simulink model "TCP_Test"  (R2024a)
settings: Solver=FixedStepAuto  StartTime=0.0  StopTime=10.0  RelTol=1e-3  EnableMultiTasking=on
libraries: px4Sensorslib x1, px4Utilslib x1
settings Model: ExtModeTrigDuration=10  Creator=root  LastModifiedBy=root
settings SolverCC: PositivePriorityOrder=on
settings OptimizationCC: OptimizeBlockIOStorage=off  BufferReuse=off  ReuseModelBlockBuffer=off  GlobalBufferReuse=off  ExpressionFolding=off  EnableMemcpy=off  PassReuseOutputArgsAs=Individual arguments  LocalBlockOutputs=off  ZeroExternalMemoryAtStartup=off  ZeroInternalMemoryAtStartup=off  MaxStackSize=64  OptimizeDataStoreBuffers=off  BusAssignmentInplaceUpdate=off  OptimizationLevel=level0  OptimizationCustomize=off  EfficientTunableParamExpr=on
settings DebuggingCC: ParameterTunabilityLossMsg=error
settings HardwareCC: ProdBitPerPointer=32  ProdBitPerSizeT=32  ProdBitPerPtrDiffT=32  ProdLargestAtomicInteger=Long  ProdLargestAtomicFloat=Double  ProdWordSize=32  ProdLongLongMode=on  ProdHWDeviceType=ARM Compatible->ARM Cortex
settings SFSimCC: SimUserSources=tcp_send.c  SimUserIncludeDirs=/home/judson/Desktop/Pixhawk/MATLAB/TCP_Test  MATLABDynamicMemAlloc=off  SimTargetLang=C++
settings SFSimCC: SimCustomHeaderCode=|
  | #include "tcp_send.h"
  | #include <netinet/in.h>
  | #include <sys/types.h>
  | #include <sys/socket.h>
  | #include <arpa/inet.h>
  | #include <errno.h>
  | #include <stdio.h>
  | #include <string.h>
  | #include <unistd.h>
settings RTWCC: Description=Embedded Coder  SystemTargetFile=ert.tlc  HardwareBoard=PX4 Pixhawk 6x  TLCOptions="-aInlineSetEventsForThisBaseRateFcn=TLC_FALSE -aSuppressMultiTaskScheduler=TLC_FALSE  -aRateBasedStepFcn=0"  TemplateMakefile=ert_default_tmf  RTWUseSimCustomCode=on  CustomInclude=/home/judson/Desktop/Pixhawk/MATLAB/TCP_Test  CustomSource=tcp_send.c  Toolchain=GNU Tools for PX4 Autopilots  BuildConfiguration=Debug  TargetLang=C++
settings RTWCC: CustomHeaderCode=|
  | #include "tcp_send.h"
  | #include <netinet/in.h>
  | #include <sys/types.h>
  | #include <sys/socket.h>
  | #include <arpa/inet.h>
  | #include <errno.h>
  | #include <stdio.h>
  | #include <string.h>
  | #include <unistd.h>
settings CodeAppCC: ForceParamTrailComments=on  IgnoreCustomStorageClasses=off  OperatorAnnotations=on  SimulinkDataObjDesc=on  SFDataObjDesc=on  MATLABFcnDesc=on  InsertBlockDesc=on  MATLABSourceComments=on  EnableCustomComments=on  ReqsInCode=on
settings ERTTargetCC: TargetLangStandard=C++11 (ISO)  SupportNonFinite=off  ExtModeTransport=3  ExtModeStaticAlloc=on  ExtModeStaticAllocSize=1024  ExtModeMexFile=ext_xcp  ExtModeIntrfLevel=Level2 - Open  PreserveIfCondition=on

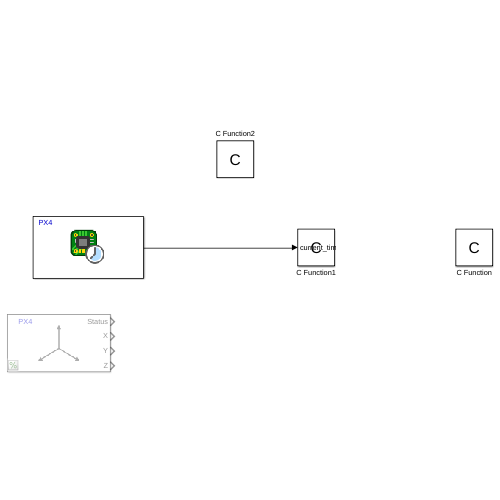
[thumbnail: Simulink's stored preview of the top-level diagram]
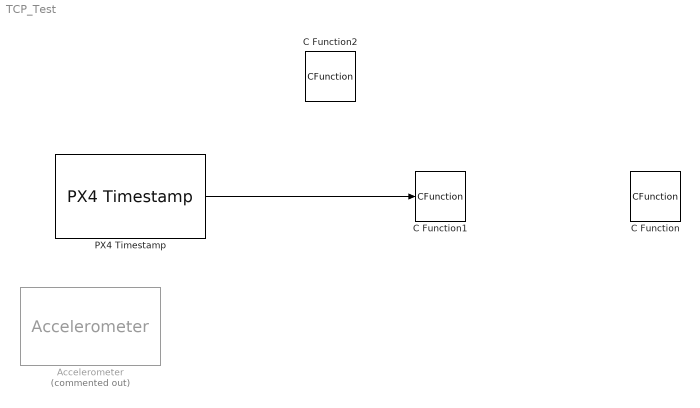
== system TCP_Test ==
  Accelerometer : px4Sensorslib/Accelerometer  Commented=on  uorbTimeStamp=off  BlockingMode=off  BlockTimeout=1e-3  sampleTime=5
  C Function : CFunction  OutputCode=|  CodegenOutputCode=|  SampleTime=0.7
      | int sock = socket(AF_INET, SOCK_DGRAM, 0);
      | 
      | struct sockaddr_in server_addr;
      | memset(&server_addr, 0, sizeof(server_addr));
      | server_addr.sin_family = AF_INET;
      | server_addr.sin_port = htons(8080);
      | 
      | if (inet_pton(AF_INET, "192.168.0.210", &server_addr.sin_addr) <= 0) {
      |   close(sock);
      | }
      | 
      | 
      | int result = connect(sock, (struct sockaddr*)&server_addr, sizeof(server_addr));
      | if (result < 0) {
      |   close(sock);
      | }
      | 
      | char message[] = "Hello from PX4 very fast!";
      | send(sock, message, strlen(message), 0);
      | 
      | close(sock);
      | int sock = socket(AF_INET, SOCK_DGRAM, 0);
      | 
      | struct sockaddr_in server_addr;
      | memset(&server_addr, 0, sizeof(server_addr));
      | server_addr.sin_family = AF_INET;
      | server_addr.sin_port = htons(8080);
      | 
      | if (inet_pton(AF_INET, "192.168.0.210", &server_addr.sin_addr) <= 0) {
      |   close(sock);
      | }
      | 
      | 
      | int result = connect(sock, (struct sockaddr*)&server_addr, sizeof(server_addr));
      | if (result < 0) {
      |   close(sock);
      | }
      | 
      | char message[] = "Hello from PX4 very fast!";
      | send(sock, message, strlen(message), 0);
      | 
      | close(sock);
  C Function1 : CFunction  OutputCode=|  CodegenOutputCode=|
      | int sock = socket(AF_INET, SOCK_DGRAM, 0);
      |     if (sock < 0) {
      |         return;  // Failed to create socket
      |     }
      | 
      |     struct sockaddr_in server_addr;
      |     memset(&server_addr, 0, sizeof(server_addr));
      |     server_addr.sin_family = AF_INET;
      |     server_addr.sin_port = htons(8080);
      |     server_addr.sin_addr.s_addr = inet_addr("192.168.0.129");
      | 
      |     // Convert uint64 to a char array (string)
      |     char message[32];
      |     snprintf(message, sizeof(message), "%llu", (unsigned long long) current_time);  // Convert to string
      | 
      |     // Send the formatted string over UDP
      |     sendto(sock, message, strlen(message), 0, (struct sockaddr*)&server_addr, sizeof(server_addr));
      | 
      |     close(sock);
      | int sock = socket(AF_INET, SOCK_DGRAM, 0);
      |     if (sock < 0) {
      |         return;  // Failed to create socket
      |     }
      | 
      |     struct sockaddr_in server_addr;
      |     memset(&server_addr, 0, sizeof(server_addr));
      |     server_addr.sin_family = AF_INET;
      |     server_addr.sin_port = htons(8080);
      |     server_addr.sin_addr.s_addr = inet_addr("192.168.0.129");
      | 
      |     // Convert uint64 to a char array (string)
      |     char message[32];
      |     snprintf(message, sizeof(message), "%llu", (unsigned long long) current_time);  // Convert to string
      | 
      |     // Send the formatted string over UDP
      |     sendto(sock, message, strlen(message), 0, (struct sockaddr*)&server_addr, sizeof(server_addr));
      | 
      |     close(sock);
  C Function2 : CFunction  OutputCode=|  CodegenOutputCode=|  SampleTime=30  SimCustomHeaderFile=#include <unistd.h> // For usleep()  CustomHeaderFile=#include <unistd.h> // For usleep()
      OutputCode=|
      | // uint64_T initial_time;
      | // uint64_T current_time;
      | 
      | // initial_time = hrt_absolute_time();
      | // current_time = hrt_absolute_time();
      | 
      | // while (current_time - 10000000 < initial_time) {
      | //     
      | // }
      | int sock = socket(AF_INET, SOCK_DGRAM, 0);
      | 
      | struct sockaddr_in server_addr;
      | memset(&server_addr, 0, sizeof(server_addr));
      | server_addr.sin_family = AF_INET;
      | server_addr.sin_port = htons(8080);
      | 
      | if (inet_pton(AF_INET, "192.168.0.129", &server_addr.sin_addr) <= 0) {
      |   close(sock);
      | }
      | 
      | 
      | int result = connect(sock, (struct sockaddr*)&server_addr, sizeof(server_addr));
      | if (result < 0) {
      |   close(sock);
      | }
      | 
      | char message[] = "Sleeping for 10s";
      | send(sock, message, strlen(message), 0);
      | 
      | 
      | 
      | //usleep(10 * 1000000);
      | 
      | uint64_t start_time = hrt_absolute_time();  // Get current time in microseconds
      | while (hrt_absolute_time() - start_time < 10 * 1000000) {
      | // Do nothing, just waste CPU cycles
      | }
      | 
      | 
      | char message2[] = "Awakened after 10s";
      | send(sock, message2, strlen(message2), 0);
      | 
      | close(sock);
      CodegenOutputCode=|
      | // uint64_T initial_time;
      | // uint64_T current_time;
      | 
      | // initial_time = hrt_absolute_time();
      | // current_time = hrt_absolute_time();
      | 
      | // while (current_time - 10000000 < initial_time) {
      | //     
      | // }
      | int sock = socket(AF_INET, SOCK_DGRAM, 0);
      | 
      | struct sockaddr_in server_addr;
      | memset(&server_addr, 0, sizeof(server_addr));
      | server_addr.sin_family = AF_INET;
      | server_addr.sin_port = htons(8080);
      | 
      | if (inet_pton(AF_INET, "192.168.0.129", &server_addr.sin_addr) <= 0) {
      |   close(sock);
      | }
      | 
      | 
      | int result = connect(sock, (struct sockaddr*)&server_addr, sizeof(server_addr));
      | if (result < 0) {
      |   close(sock);
      | }
      | 
      | char message[] = "Sleeping for 10s";
      | send(sock, message, strlen(message), 0);
      | 
      | 
      | 
      | //usleep(10 * 1000000);
      | 
      | uint64_t start_time = hrt_absolute_time();  // Get current time in microseconds
      | while (hrt_absolute_time() - start_time < 10 * 1000000) {
      | // Do nothing, just waste CPU cycles
      | }
      | 
      | 
      | char message2[] = "Awakened after 10s";
      | send(sock, message2, strlen(message2), 0);
      | 
      | close(sock);
  PX4 Timestamp : px4Utilslib/PX4 Timestamp  SampleTime=1
      settings: SourceProductName=PX4 Utility Blocks
  wires:
  PX4 Timestamp/1 -> C Function1/1
